simulink model "sys_model"  (R2020b)
settings: Solver=VariableStepAuto  StartTime=0.0  StopTime=10.0  RelTol=1e-3
undefined symbols (not defined in the file): be, bv, Ie, Iv
settings Model: Creator=Rasika Shejul  LastModifiedBy=Rushikesh

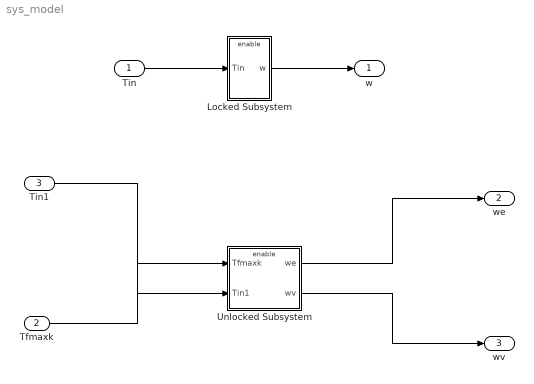
== system sys_model ==
  Tin : Inport
  Tfmaxk : Inport  Port=2
  Tin1 : Inport  Port=3
  Locked Subsystem : Subsystem
  Unlocked Subsystem : Subsystem
  w : Outport  InitialOutput=0  VectorParamsAs1DForOutWhenUnconnected=off
  we : Outport  Port=2  InitialOutput=0  VectorParamsAs1DForOutWhenUnconnected=off
  wv : Outport  Port=3  InitialOutput=0  VectorParamsAs1DForOutWhenUnconnected=off
  wires:
  Locked Subsystem/1(w) -> w/1
  Unlocked Subsystem/2(wv) -> wv/1
  Tin1/1 -> Unlocked Subsystem/2(Tin1)
  Unlocked Subsystem/1(we) -> we/1
  Tin/1 -> Locked Subsystem/1(Tin)
  Tfmaxk/1 -> Unlocked Subsystem/1(Tfmaxk)

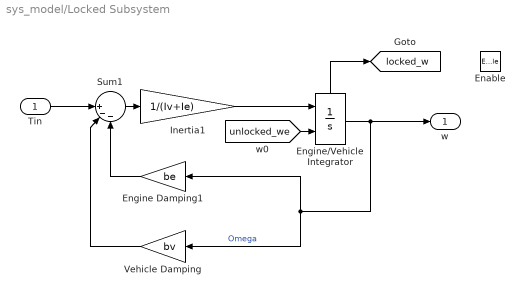
== system sys_model/Locked Subsystem ==
  Tin : Inport
  Enable : EnablePort
  Engine Damping1 : Gain  Gain=be  SaturateOnIntegerOverflow=on  OutDataTypeStr=Inherit: Same as input  ParamDataTypeStr=Inherit: Same as input
  Engine/Vehicle Integrator : Integrator  InitialConditionSource=external  ShowStatePort=on
  Inertia1 : Gain  Gain=1/(Iv+Ie)  SaturateOnIntegerOverflow=on  OutDataTypeStr=Inherit: Same as input  ParamDataTypeStr=Inherit: Same as input
  Sum1 : Sum  Inputs=||+--  InputSameDT=on  SaturateOnIntegerOverflow=on  OutDataTypeStr=Inherit: Same as first input
  Vehicle Damping : Gain  Gain=bv  SaturateOnIntegerOverflow=on  OutDataTypeStr=Inherit: Same as input  ParamDataTypeStr=Inherit: Same as input
  w : Outport  InitialOutput=0  VectorParamsAs1DForOutWhenUnconnected=off
  tag scope: locked_w=global
  wires:
  Engine Damping1/1 -> Sum1/3
  Engine/Vehicle Integrator/1 -> w/1, Engine Damping1/1, Vehicle Damping/1  "Omega"
  [unlocked_we] -> Engine/Vehicle Integrator/2
  Sum1/1 -> Inertia1/1
  Tin/1 -> Sum1/1
  Vehicle Damping/1 -> Sum1/2
  Engine/Vehicle Integrator/State -> [locked_w]
  Inertia1/1 -> Engine/Vehicle Integrator/1

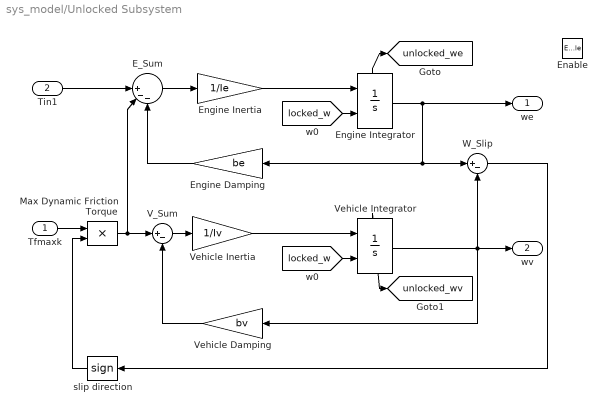
== system sys_model/Unlocked Subsystem ==
  Tfmaxk : Inport
  Tin1 : Inport  Port=2
  Enable : EnablePort
  E_Sum : Sum  Inputs=||+--  InputSameDT=on  SaturateOnIntegerOverflow=on  OutDataTypeStr=Inherit: Same as first input
  Engine Damping : Gain  Gain=be  SaturateOnIntegerOverflow=on  OutDataTypeStr=Inherit: Same as input  ParamDataTypeStr=Inherit: Same as input
  Engine Inertia : Gain  Gain=1/Ie  SaturateOnIntegerOverflow=on  OutDataTypeStr=Inherit: Same as input  ParamDataTypeStr=Inherit: Same as input
  Engine Integrator : Integrator  InitialConditionSource=external  ShowStatePort=on
  Max Dynamic Friction Torque : Product  InputSameDT=on  RndMeth=Zero  SaturateOnIntegerOverflow=on  OutDataTypeStr=Inherit: Same as first input
  V_Sum : Sum  Inputs=|+-  InputSameDT=on  SaturateOnIntegerOverflow=on  OutDataTypeStr=Inherit: Same as first input
  Vehicle Damping : Gain  Gain=bv  SaturateOnIntegerOverflow=on  OutDataTypeStr=Inherit: Same as input  ParamDataTypeStr=Inherit: Same as input
  Vehicle Inertia : Gain  Gain=1/Iv  SaturateOnIntegerOverflow=on  OutDataTypeStr=Inherit: Same as input  ParamDataTypeStr=Inherit: Same as input
  Vehicle Integrator : Integrator  InitialConditionSource=external  ShowStatePort=on
  W_Slip : Sum  Inputs=|+-  InputSameDT=on  SaturateOnIntegerOverflow=on  OutDataTypeStr=Inherit: Same as first input
  slip direction : Signum
  we : Outport  InitialOutput=0  VectorParamsAs1DForOutWhenUnconnected=off
  wv : Outport  Port=2  InitialOutput=0  VectorParamsAs1DForOutWhenUnconnected=off
  tag scope: unlocked_we=global, unlocked_wv=global
  wires:
  E_Sum/1 -> Engine Inertia/1
  Vehicle Integrator/1 -> wv/1, W_Slip/2, Vehicle Damping/1
  Vehicle Integrator/State -> [unlocked_wv]
  Engine Integrator/1 -> we/1, Engine Damping/1, W_Slip/1
  Vehicle Inertia/1 -> Vehicle Integrator/1
  [locked_w] -> Vehicle Integrator/2
  Tfmaxk/1 -> Max Dynamic Friction Torque/1
  W_Slip/1 -> slip direction/1
  Engine Inertia/1 -> Engine Integrator/1
  Vehicle Damping/1 -> V_Sum/2
  V_Sum/1 -> Vehicle Inertia/1
  slip direction/1 -> Max Dynamic Friction Torque/2
  [locked_w] -> Engine Integrator/2
  Max Dynamic Friction Torque/1 -> V_Sum/1, E_Sum/2
  Tin1/1 -> E_Sum/1
  Engine Integrator/State -> [unlocked_we]
  Engine Damping/1 -> E_Sum/3
